simulink model "multi__micro1nosw_droop"  (R2015a)
settings: Solver=ode23tb  StartTime=0.0  StopTime=2
model workspace: external: MAT-File D:\google drive\project\nn1\matla.mat (data not in the file)
undefined symbols (not defined in the file): cf, gam, gamp, k1, k2, k3, k5, Lc, lf, mp1, mp2, Mu, nq1, nq2, rc, sig, sigp, td, wn
libraries: powerlib x113, simulink x32, powerlib_meascontrol x32, powerlib_extras x2
(part 5 of 5)

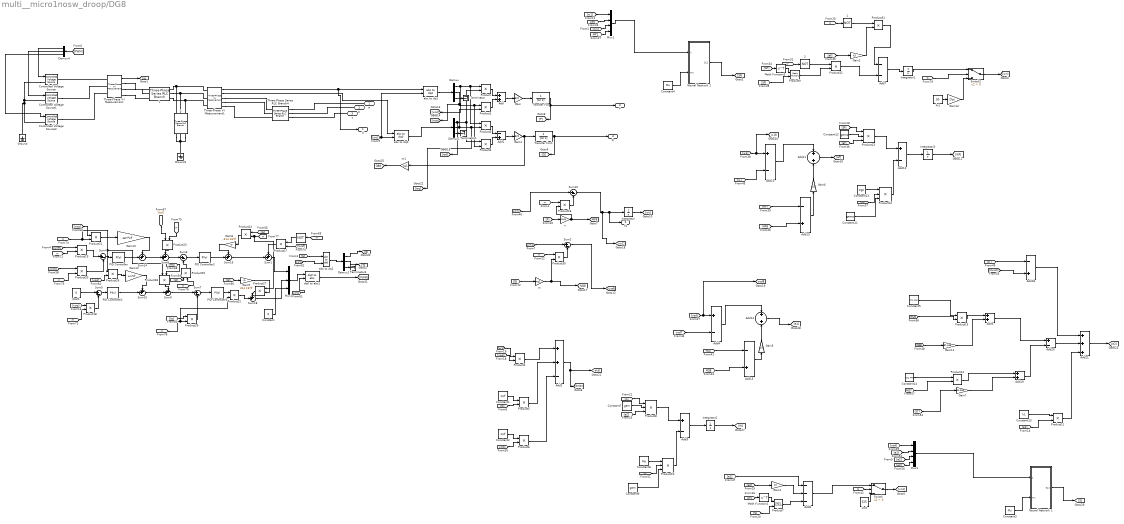
== system multi__micro1nosw_droop/DG8 ==
  " " : Logic  Operator=NOT  AllPortsSameDT=off  OutDataTypeStr=boolean
  " 1" : Logic  Operator=NOT  AllPortsSameDT=off  OutDataTypeStr=boolean
  " 2" : Logic  Operator=NOT  AllPortsSameDT=off  OutDataTypeStr=boolean
  Add{,5,11,14,19} (5 alike) : Sum
  Add{1,13,15,18} (4 alike) : Sum  Inputs=-+
  Add{4,9..10,12,20} (5 alike) : Sum  Inputs=+-
  Add2 : Sum  Inputs=++-
  Add21 : Sum  Inputs=+++
  Add7 : Sum  Inputs=--
  Add8 : Sum  Inputs=---
  C : powerlib/Elements/Three-Phase Series RLC Branch  LConnTagsString=A|B|C  RConnTagsString=A|B|C  BranchType=C  Resistance=1  Inductance=1e-3  Capacitance=cf  Measurements=None
  Constant : Constant  Value=0
  Constant1 : Constant  Value=1/cf
  Constant11 : Constant  Value=gamp
  Constant12 : Constant  Value=gamp
  Constant13 : Constant  Value=sigp
  Constant14 : Constant  Value=-31.446
  Constant15 : Constant  Value=k1
  Constant2 : Constant  Value=1/cf
  Constant3 : Constant  Value=Mu
  Constant4 : Constant  Value=Mu
  Constant5 : Constant  Value=-31.446
  Constant7 : Constant  Value=gam
  Constant8 : Constant  Value=sig
  Constant9 : Constant  Value=gam
  Controlled Voltage Source : powerlib/Electrical Sources/Controlled Voltage Source  Initialize=off  Source_Type=AC  Amplitude=325  Phase=0  Frequency=50  Measurements=None
  Controlled Voltage Source1 : powerlib/Electrical Sources/Controlled Voltage Source  Initialize=off  Source_Type=AC  Amplitude=325  Phase=0  Frequency=50  Measurements=None
  Controlled Voltage Source2 : powerlib/Electrical Sources/Controlled Voltage Source  Initialize=off  Source_Type=AC  Amplitude=325  Phase=0  Frequency=50  Measurements=None
  Demux{,1..2,4} (4 alike) : Demux  Outputs=3
  Gain : Gain  Gain=3/2
  Gain1 : Gain  Gain=3/2
  Gain10 : Gain  Gain=-wn*cf
  Gain11 : Gain  Gain=31.446
  Gain12 : Gain  Gain=wn*cf
  Gain13 : Gain  Gain=2*pi
  Gain2 : Gain  Gain=k3
  Gain4 : Gain  Gain=k2
  Gain5 : Gain  Gain=k5
  Gain6 : Gain  Gain=k5
  Gain7 : Gain  Gain=31.446
  Gain8 : Gain  Gain=-314.16*lf
  Gain9 : Gain  Gain=314.16*lf
  Ground : powerlib/Elements/Ground  LConnTagsString=a
  Ground1 : powerlib/Elements/Ground  LConnTagsString=a
  Integrator : Integrator  UpperSaturationLimit=314.16  ZeroCross=off
  Integrator1 : Integrator  InitialCondition=wn-1  UpperSaturationLimit=321  LowerSaturationLimit=314.16
  Integrator2 : Integrator  InitialCondition=zeros(16.,1)  UpperSaturationLimit=314.16  ZeroCross=off
  Integrator3 : Integrator  InitialCondition=zeros(16,1)  UpperSaturationLimit=314.16  ZeroCross=off
  L : powerlib/Elements/Three-Phase Series RLC Branch  LConnTagsString=A|B|C  RConnTagsString=A|B|C  BranchType=RL  Resistance=0.1  Inductance=lf  Capacitance=1e-6  Measurements=None
  Math Function1 : Math  Operator=transpose  OutputSignalType=real  SaturateOnIntegerOverflow=on
  Math Function3 : Math  Operator=transpose  OutputSignalType=real  SaturateOnIntegerOverflow=on
  Mux1 : Mux
  Mux2 : Mux  Inputs=3
  Mux3 : Mux
  Neural Network 1 : MATLAB Function  TreatAsAtomicUnit=on
  Neural Network 2 : MATLAB Function  TreatAsAtomicUnit=on
  PID Controller : simulink/Continuous/PID Controller  Controller=PI  TimeDomain=Continuous-time  SampleTime=-1  IntegratorMethod=Forward Euler  FilterMethod=Forward Euler  Form=Parallel  UseFilter=on  ControllerParametersSource=internal  P=0.1  I=420  D=0  N=0  InitialConditionSource=internal  InitialConditionForIntegrator=0  InitialConditionForFilter=0  ExternalReset=none  LimitOutput=off  UpperSaturationLimit=inf  LowerSaturationLimit=-inf  LinearizeAsGain=on  AntiWindupMode=none  Kb=1  TrackingMode=off  Kt=1  PParamMin=[]  PParamMax=[]  IParamMin=[]  IParamMax=[]  DParamMin=[]  DParamMax=[]  NParamMin=[]  NParamMax=[]  KbParamMin=[]  KbParamMax=[]  KtParamMin=[]  KtParamMax=[]  POutMin=[]  POutMax=[]  IOutMin=[]  IOutMax=[]  DOutMin=[]  DOutMax=[]  NOutMin=[]  NOutMax=[]  KbOutMin=[]  KbOutMax=[]  KtOutMin=[]  KtOutMax=[]  IntegratorOutMin=[]  IntegratorOutMax=[]  FilterOutMin=[]  FilterOutMax=[]  SumOutMin=[]  SumOutMax=[]  SumI1OutMin=[]  SumI1OutMax=[]  SumI2OutMin=[]  SumI2OutMax=[]  SumI3OutMin=[]  SumI3OutMax=[]  SumDOutMin=[]  SumDOutMax=[]  SaturationOutMin=[]  SaturationOutMax=[]  IntegratorContinuousStateAttributes=''  IntegratorStateMustResolveToSignalObject=off  IntegratorRTWStateStorageClass=Auto  FilterContinuousStateAttributes=''  FilterStateMustResolveToSignalObject=off  FilterRTWStateStorageClass=Auto  DifferentiatorICPrevScaledInput=0  DifferentiatorOutMin=[]  DifferentiatorOutMax=[]
  PID Controller1 : simulink/Continuous/PID Controller  Controller=PI  TimeDomain=Continuous-time  SampleTime=-1  IntegratorMethod=Forward Euler  FilterMethod=Forward Euler  Form=Parallel  UseFilter=on  ControllerParametersSource=internal  P=0.1  I=420  D=0  N=0  InitialConditionSource=internal  InitialConditionForIntegrator=0  InitialConditionForFilter=0  ExternalReset=none  LimitOutput=off  UpperSaturationLimit=inf  LowerSaturationLimit=-inf  LinearizeAsGain=on  AntiWindupMode=none  Kb=1  TrackingMode=off  Kt=1  PParamMin=[]  PParamMax=[]  IParamMin=[]  IParamMax=[]  DParamMin=[]  DParamMax=[]  NParamMin=[]  NParamMax=[]  KbParamMin=[]  KbParamMax=[]  KtParamMin=[]  KtParamMax=[]  POutMin=[]  POutMax=[]  IOutMin=[]  IOutMax=[]  DOutMin=[]  DOutMax=[]  NOutMin=[]  NOutMax=[]  KbOutMin=[]  KbOutMax=[]  KtOutMin=[]  KtOutMax=[]  IntegratorOutMin=[]  IntegratorOutMax=[]  FilterOutMin=[]  FilterOutMax=[]  SumOutMin=[]  SumOutMax=[]  SumI1OutMin=[]  SumI1OutMax=[]  SumI2OutMin=[]  SumI2OutMax=[]  SumI3OutMin=[]  SumI3OutMax=[]  SumDOutMin=[]  SumDOutMax=[]  SaturationOutMin=[]  SaturationOutMax=[]  IntegratorContinuousStateAttributes=''  IntegratorStateMustResolveToSignalObject=off  IntegratorRTWStateStorageClass=Auto  FilterContinuousStateAttributes=''  FilterStateMustResolveToSignalObject=off  FilterRTWStateStorageClass=Auto  DifferentiatorICPrevScaledInput=0  DifferentiatorOutMin=[]  DifferentiatorOutMax=[]
  PID Controller2 : simulink/Continuous/PID Controller  Controller=PI  TimeDomain=Continuous-time  SampleTime=-1  IntegratorMethod=Forward Euler  FilterMethod=Forward Euler  Form=Parallel  UseFilter=on  ControllerParametersSource=internal  P=15  I=20000  D=0  N=0  InitialConditionSource=internal  InitialConditionForIntegrator=0  InitialConditionForFilter=0  ExternalReset=none  LimitOutput=off  UpperSaturationLimit=inf  LowerSaturationLimit=-inf  LinearizeAsGain=on  AntiWindupMode=none  Kb=1  TrackingMode=off  Kt=1  PParamMin=[]  PParamMax=[]  IParamMin=[]  IParamMax=[]  DParamMin=[]  DParamMax=[]  NParamMin=[]  NParamMax=[]  KbParamMin=[]  KbParamMax=[]  KtParamMin=[]  KtParamMax=[]  POutMin=[]  POutMax=[]  IOutMin=[]  IOutMax=[]  DOutMin=[]  DOutMax=[]  NOutMin=[]  NOutMax=[]  KbOutMin=[]  KbOutMax=[]  KtOutMin=[]  KtOutMax=[]  IntegratorOutMin=[]  IntegratorOutMax=[]  FilterOutMin=[]  FilterOutMax=[]  SumOutMin=[]  SumOutMax=[]  SumI1OutMin=[]  SumI1OutMax=[]  SumI2OutMin=[]  SumI2OutMax=[]  SumI3OutMin=[]  SumI3OutMax=[]  SumDOutMin=[]  SumDOutMax=[]  SaturationOutMin=[]  SaturationOutMax=[]  IntegratorContinuousStateAttributes=''  IntegratorStateMustResolveToSignalObject=off  IntegratorRTWStateStorageClass=Auto  FilterContinuousStateAttributes=''  FilterStateMustResolveToSignalObject=off  FilterRTWStateStorageClass=Auto  DifferentiatorICPrevScaledInput=0  DifferentiatorOutMin=[]  DifferentiatorOutMax=[]
  PID Controller3 : simulink/Continuous/PID Controller  Controller=PI  TimeDomain=Continuous-time  SampleTime=-1  IntegratorMethod=Forward Euler  FilterMethod=Forward Euler  Form=Parallel  UseFilter=on  ControllerParametersSource=internal  P=15  I=20000  D=0  N=0  InitialConditionSource=internal  InitialConditionForIntegrator=0  InitialConditionForFilter=0  ExternalReset=none  LimitOutput=off  UpperSaturationLimit=inf  LowerSaturationLimit=-inf  LinearizeAsGain=on  AntiWindupMode=none  Kb=1  TrackingMode=off  Kt=1  PParamMin=[]  PParamMax=[]  IParamMin=[]  IParamMax=[]  DParamMin=[]  DParamMax=[]  NParamMin=[]  NParamMax=[]  KbParamMin=[]  KbParamMax=[]  KtParamMin=[]  KtParamMax=[]  POutMin=[]  POutMax=[]  IOutMin=[]  IOutMax=[]  DOutMin=[]  DOutMax=[]  NOutMin=[]  NOutMax=[]  KbOutMin=[]  KbOutMax=[]  KtOutMin=[]  KtOutMax=[]  IntegratorOutMin=[]  IntegratorOutMax=[]  FilterOutMin=[]  FilterOutMax=[]  SumOutMin=[]  SumOutMax=[]  SumI1OutMin=[]  SumI1OutMax=[]  SumI2OutMin=[]  SumI2OutMax=[]  SumI3OutMin=[]  SumI3OutMax=[]  SumDOutMin=[]  SumDOutMax=[]  SaturationOutMin=[]  SaturationOutMax=[]  IntegratorContinuousStateAttributes=''  IntegratorStateMustResolveToSignalObject=off  IntegratorRTWStateStorageClass=Auto  FilterContinuousStateAttributes=''  FilterStateMustResolveToSignalObject=off  FilterRTWStateStorageClass=Auto  DifferentiatorICPrevScaledInput=0  DifferentiatorOutMin=[]  DifferentiatorOutMax=[]
  Product{,1,3..4} (4 alike) : Product  RndMeth=Zero
  Product{8,10,12..13} (4 alike) : Product  Inputs=3
  Product{2,5..6,11,14..32} (23 alike) : Product
  Product7 : Product  Multiplication=Matrix(*)
  Product9 : Product  Multiplication=Matrix(*)
  Qref1 : Constant  Value=0
  Sum{1,8..9,14..16,18} (7 alike) : Sum  Inputs=++|  SaturateOnIntegerOverflow=on  InputSameDT=on  OutDataTypeStr=Inherit: Same as first input
  Sum{2,4..7,10} (6 alike) : Sum  Inputs=|+-
  Switch : Switch  Criteria=u2 > Threshold
  Switch2 : Switch  Criteria=u2 > Threshold  ZeroCross=off
  Terminator : Terminator
  Terminator1 : Terminator
  Terminator4 : Terminator
  Three-Phase Series RLC Branch4 : powerlib/Elements/Three-Phase Series RLC Branch  LConnTagsString=A|B|C  RConnTagsString=A|B|C  BranchType=RL  Resistance=rc  Inductance=Lc  Capacitance=1e-6  Measurements=None
  Three-Phase V-I Measurement : powerlib/Measurements/Three-Phase V-I Measurement  VoltageMeasurement=no  SetLabelV=off  LabelV=Vabc  Vpu=off  VpuLL=off  CurrentMeasurement=yes  SetLabelI=off  LabelI=Iabc  Ipu=off  Pbase=100e6  Vbase=500e3  OutputType=Complex  PhasorSimulation=off  PSBequivalent=0
  Three-Phase V-I Measurement1 : powerlib/Measurements/Three-Phase V-I Measurement  VoltageMeasurement=phase-to-ground  SetLabelV=off  LabelV=Vabc  Vpu=off  VpuLL=off  CurrentMeasurement=yes  SetLabelI=off  LabelI=Iabc  Ipu=off  Pbase=100e6  Vbase=500e3  OutputType=Complex  PhasorSimulation=off  PSBequivalent=0
  Transfer Fcn : TransferFcn  Denominator=[td 1]
  Transfer Fcn1 : TransferFcn  Denominator=[td 1]
  Un5 : Constant  Value=325
  abc to dq0 : powerlib_meascontrol/Transformations/abc to dq0  Alignment=90 degrees behind phase A axis
  abc to dq1 : powerlib_meascontrol/Transformations/abc to dq0  Alignment=90 degrees behind phase A axis
  abc to dq2 : powerlib_meascontrol/Transformations/abc to dq0  Alignment=90 degrees behind phase A axis
  dq0 to abc1 : powerlib_meascontrol/Transformations/dq0 to abc  Alignment=90 degrees behind phase A axis
  fn1 : Constant  Value=50
  m : Gain  Gain=nq1
  m1 : Gain  Gain=nq1
  n : Gain  Gain=mp1
  a : PMIOPort  Tag=PMCPort  Port=1  Side=Right
  b : PMIOPort  Tag=PMCPort  Port=2  Side=Right
  c : PMIOPort  Tag=PMCPort  Port=3  Side=Right
  U : Outport
  f1 : Outport  Port=2
  P : Outport  Port=3
  Q : Outport  Port=4
  tag scope: MP8=global, NQ8=global, Q88=global, dv8=global, vod8=global, w18=global
  wires:
  [PWM] -> Demux4/1
  Three-Phase V-I Measurement1/1 -> U/1, abc to dq1/1
  Three-Phase V-I Measurement1/2 -> abc to dq0/1
  Demux/1 -> [vod], Product/1, Product3/1
  Demux1/1 -> [iod], Product/2, Product4/1
  Demux/2 -> [voq], Product1/1, Product4/2
  Demux1/2 -> Product1/2, [ioq], Product3/2
  Product/1 -> Add/1
  Product1/1 -> Add/2
  Product3/1 -> Add1/1
  Product4/1 -> Add1/2
  [wt] -> abc to dq1/2, abc to dq0/2
  [P] -> n/1
  Demux4/1 -> Controlled Voltage Source/1
  Demux4/2 -> Controlled Voltage Source1/1
  Demux4/3 -> Controlled Voltage Source2/1
  Three-Phase V-I Measurement/1 -> [IL]
  Add/1 -> Gain/1
  Gain/1 -> Transfer Fcn/1
  Add1/1 -> Gain1/1
  Gain1/1 -> m1/1, Transfer Fcn1/1
  abc to dq1/1 -> Demux/1
  abc to dq0/1 -> Demux1/1
  [wn] -> Sum10/1
  Integrator/1 -> [wt]
  [w1] -> Product2/1
  [voq] -> Product2/2
  Product2/1 -> Add2/1
  Constant1/1 -> Product5/1
  [Id] -> Product5/2
  Product5/1 -> Add2/2
  Constant2/1 -> Product6/1
  [iod] -> Product6/2
  Product6/1 -> Add2/3
  Add2/1 -> [dvodi], [dv8]
  Demux/3 -> Terminator/1
  Demux1/3 -> Terminator1/1
  [Q] -> m/1
  Sum2/1 -> [Uref]
  Gain4/1 -> Add8/2
  [e2] -> Gain4/1
  [S] -> Product7/2
  [W] -> Math Function1/1
  Math Function1/1 -> Product7/1
  Product7/1 -> Add8/3
  [S] -> Product8/1
  Constant7/1 -> Product8/2
  [e2] -> Product8/3
  Product8/1 -> Add9/1
  Constant8/1 -> Product10/1
  [W] -> Product10/2
  Product10/1 -> Add9/2
  Constant9/1 -> Product10/3
  Add9/1 -> Integrator2/1
  Integrator2/1 -> [W]
  Transfer Fcn/1 -> P/1, [P]
  Transfer Fcn1/1 -> Q/1, [Q]
  [Sf] -> Product13/1
  Constant12/1 -> Product13/2
  [ef] -> Product13/3
  Product13/1 -> Add12/1
  Constant13/1 -> Product12/1
  [Wf] -> Product12/2
  Product12/1 -> Add12/2
  Constant11/1 -> Product12/3
  Add12/1 -> Integrator3/1
  Integrator3/1 -> [Wf]
  [w1] -> Mux1/1
  [ef] -> Mux1/2
  [wn] -> Mux1/3
  [MP1] -> Mux1/4
  [w1] -> [w18], Add10/1
  [w17] -> Add10/2
  Add10/1 -> Add11/1
  [MP7] -> Add13/1
  [MP8] -> Add13/2
  Add13/1 -> Gain6/1
  Add11/1 -> [ef]
  [vod] -> [vod8], Add4/1
  [vod7] -> Add4/2
  Add4/1 -> Add14/1
  [NQ7] -> Add15/1
  [NQ8] -> Add15/2
  Add15/1 -> Gain5/1
  Add14/1 -> [e1]
  Gain5/1 -> Add14/2
  Gain6/1 -> Add11/2
  [e1] -> Add8/1
  m1/1 -> [Q88]
  [vod] -> Mux3/1
  [e1] -> Mux3/2
  [e2] -> Mux3/3
  [e2] -> Mux3/4
  Constant5/1 -> Product15/1
  [NQ8] -> Product15/2
  Product15/1 -> Add5/1
  [Q88] -> Gain11/1
  Constant14/1 -> Product14/1
  [NQ7] -> Product14/2
  Product14/1 -> Add19/1
  [Q77] -> Gain7/1
  Add19/1 -> Add20/2
  Add5/1 -> Add20/1
  Gain7/1 -> Add19/2
  Gain11/1 -> Add5/2
  Add20/1 -> Add21/2
  Constant15/1 -> Product11/1
  [e1] -> Product11/2
  Product11/1 -> Add21/3
  [dv7] -> Add18/1
  Add18/1 -> Add21/1
  Add21/1 -> [e2]
  [dvodi] -> Add18/2
  [IL] -> abc to dq2/1
  Demux2/1 -> [Id]
  Demux2/2 -> [Iq]
  [wt] -> abc to dq2/2
  Qref1/1 -> Sum5/1
  Sum4/1 -> PID Controller/1
  Sum5/1 -> PID Controller1/1
  Sum18/1 -> Mux2/2
  Constant/1 -> Mux2/3
  PID Controller/1 -> Sum14/2
  PID Controller1/1 -> Sum15/2
  Gain10/1 -> Sum14/1
  Gain12/1 -> Sum15/1
  Sum15/1 -> Sum9/2
  Sum9/1 -> Sum7/1
  Sum14/1 -> Sum8/2
  Sum8/1 -> Sum6/1
  Sum6/1 -> PID Controller2/1
  Sum7/1 -> PID Controller3/1
  Gain8/1 -> Sum16/1
  PID Controller2/1 -> Sum16/2
  [Id] -> Gain9/1
  Mux2/1 -> dq0 to abc1/1
  [wt] -> dq0 to abc1/2
  abc to dq2/1 -> Demux2/1
  dq0 to abc1/1 -> [PWM]
  Demux2/3 -> Terminator4/1
  Sum16/1 -> Sum1/2
  Sum1/1 -> Mux2/1
  Product17/1 -> Sum1/1
  [rr] -> " "/1
  [Uref] -> Product17/2
  " "/1 -> Product17/1
  [voq] -> Product18/1
  Product18/1 -> Sum5/2
  [rr] -> Product18/2
  [Uref] -> Product19/1
  Product19/1 -> Sum4/1
  [rr] -> Product19/2
  [vod] -> Product20/1
  Product20/1 -> Sum4/2
  [rr] -> Product20/2
  Product21/1 -> Gain10/1
  [voq] -> Product21/1
  [rr] -> Product28/1, Product26/1, Product21/2
  [iod] -> Product23/1
  [rr] -> Product23/2
  Product23/1 -> Sum8/1
  [Id] -> Product25/1
  Product25/1 -> Sum6/2
  [rr] -> Product25/2
  Product24/1 -> Gain8/1
  [Iq] -> Product24/1
  [rr] -> Product27/1, Product24/2
  [vod] -> Product26/2
  Product26/1 -> Gain12/1
  [ioq] -> Product28/2
  Product28/1 -> Sum9/1
  [Iq] -> Product29/1
  Product29/1 -> Sum7/2
  [rr] -> Product22/2, Product29/2
  Product27/1 -> Sum18/1
  Gain9/1 -> Product27/2
  PID Controller3/1 -> Product22/1
  Product22/1 -> Sum18/2
  [ti] -> Switch/2
  Un5/1 -> Switch/3
  Add8/1 -> Switch/1
  Switch/1 -> [vn1]
  n/1 -> [MP8], Product16/2
  Product16/1 -> Sum10/2
  [rr] -> Product16/1
  Sum10/1 -> [w1], f1/1, Integrator/1
  m/1 -> Product30/2, [NQ8]
  Product30/1 -> Sum2/2
  [rr] -> Product30/1
  [vn1] -> Sum2/1
  [Sf] -> Product9/2
  [Wf] -> Math Function3/1
  Math Function3/1 -> Product9/1
  Add7/1 -> Integrator1/1
  [ti] -> Switch2/2
  Gain13/1 -> Switch2/3
  Switch2/1 -> [wn]
  fn1/1 -> Gain13/1
  [ef] -> Gain2/1
  [rr] -> " 1"/1
  Gain2/1 -> Product31/2
  " 1"/1 -> Product31/1
  Product31/1 -> Add7/1
  [rr] -> " 2"/1
  Product9/1 -> Product32/2
  " 2"/1 -> Product32/1
  Product32/1 -> Add7/2
  Integrator1/1 -> Switch2/1
  Neural Network 1/1(Sz1) -> [S]
  Constant3/1 -> Neural Network 1/2(mu)
  Mux3/1 -> Neural Network 1/1(X)
  Neural Network 2/1(Sz1) -> [Sf]
  Constant4/1 -> Neural Network 2/2(mu)
  Mux1/1 -> Neural Network 2/1(X)
  connections:
  C/RConn1 -- Ground1/LConn1 -- C/RConn3 -- C/RConn2
  L/RConn2 -- Three-Phase V-I Measurement1/LConn2 -- C/LConn2
  L/RConn1 -- Three-Phase V-I Measurement1/LConn1 -- C/LConn1
  L/RConn3 -- Three-Phase V-I Measurement1/LConn3 -- C/LConn3
  Controlled Voltage Source/LConn1 -- Controlled Voltage Source1/LConn1 -- Ground/LConn1 -- Controlled Voltage Source2/LConn1
  Three-Phase V-I Measurement/LConn1 -- Controlled Voltage Source/RConn1
  Controlled Voltage Source1/RConn1 -- Three-Phase V-I Measurement/LConn2
  Controlled Voltage Source2/RConn1 -- Three-Phase V-I Measurement/LConn3
  Three-Phase V-I Measurement/RConn1 -- L/LConn1
  Three-Phase V-I Measurement/RConn2 -- L/LConn2
  Three-Phase V-I Measurement/RConn3 -- L/LConn3
  Three-Phase V-I Measurement1/RConn1 -- Three-Phase Series RLC Branch4/RConn1
  Three-Phase V-I Measurement1/RConn2 -- Three-Phase Series RLC Branch4/RConn2
  Three-Phase V-I Measurement1/RConn3 -- Three-Phase Series RLC Branch4/RConn3
  Three-Phase Series RLC Branch4/LConn1 -- a/RConn1
  Three-Phase Series RLC Branch4/LConn2 -- b/RConn1
  Three-Phase Series RLC Branch4/LConn3 -- c/RConn1

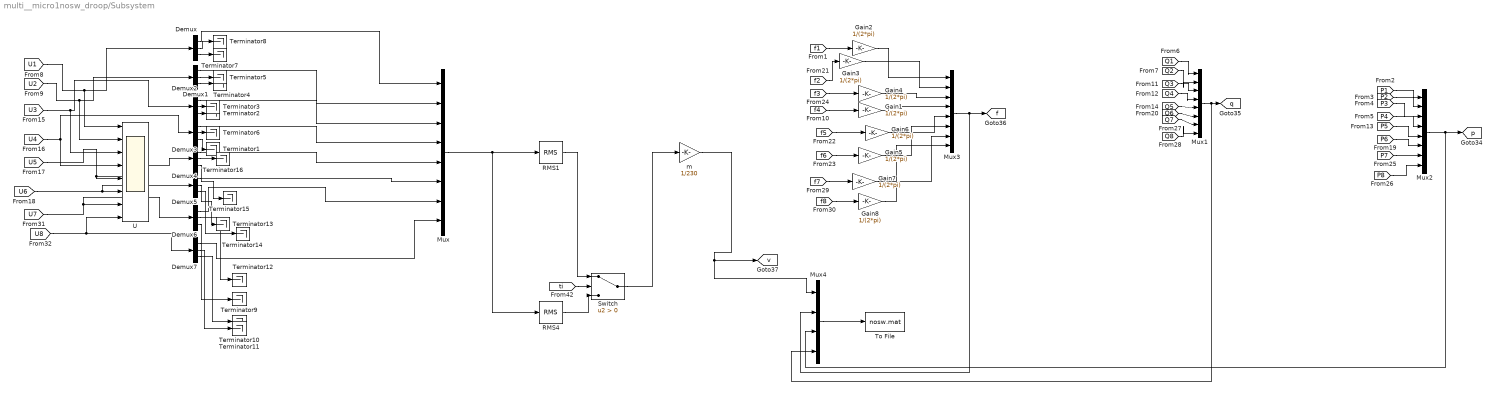
== system multi__micro1nosw_droop/Subsystem ==
  Demux{,1..7} (8 alike) : Demux  Outputs=3
  Gain{1..8} (8 alike) : Gain  Gain=1/(2*pi)
  Mux{,1..3} (4 alike) : Mux  Inputs=8
  Mux4 : Mux
  RMS1 : powerlib_extras/Measurements/RMS  f1=50
  RMS4 : powerlib_extras/Measurements/RMS  f1=49.75
  Switch : Switch  Criteria=u2 > Threshold
  Terminator{1..16} (16 alike) : Terminator
  To File : ToFile  Filename=nosw.mat  MatrixName=case1  SaveFormat=Timeseries
  U : Scope  NumInputPorts=8
      settings: TimeRange=1  YMin=-400~-400~-400~-1~-1~-1~-1~-1  YMax=400~400~400~1~1~1~1~1  SaveName=U
  m : Gain  Gain=1/230
  tag scope: f=global, p=global, q=global, v=global
  wires:
  [U6] -> Demux5/1, U/6
  Demux3/3 -> Terminator1/1
  Demux2/1 -> Mux/3
  [U5] -> Demux4/1, U/5
  Demux3/2 -> Terminator6/1
  Demux1/1 -> Mux/2
  [U4] -> Demux3/1, U/4
  Demux3/1 -> Mux/4
  Demux4/1 -> Mux/5
  Demux5/1 -> Mux/6
  Demux/3 -> Terminator7/1
  Demux2/2 -> Terminator3/1
  Demux1/3 -> Terminator4/1
  Demux1/2 -> Terminator5/1
  [U2] -> Demux1/1, U/2
  Demux/2 -> Terminator8/1
  [U3] -> Demux2/1, U/3
  [U1] -> Demux/1, U/1
  Demux2/3 -> Terminator2/1
  [U7] -> U/7, Demux6/1
  Demux7/1 -> Mux/8
  Demux6/2 -> Terminator12/1
  Demux6/3 -> Terminator9/1
  Demux5/2 -> Terminator13/1
  Demux7/2 -> Terminator11/1
  Demux4/3 -> Terminator15/1
  Demux5/3 -> Terminator14/1
  [U8] -> Demux7/1, U/8
  Demux7/3 -> Terminator10/1
  Demux4/2 -> Terminator16/1
  m/1 -> Mux4/1, [v]
  [f4] -> Gain1/1
  [f1] -> Gain2/1
  Gain1/1 -> Mux3/4
  [f3] -> Gain4/1
  [f5] -> Gain6/1
  [f6] -> Gain5/1
  Gain2/1 -> Mux3/1
  [f2] -> Gain3/1
  Gain3/1 -> Mux3/2
  Gain4/1 -> Mux3/3
  Gain5/1 -> Mux3/6
  Gain6/1 -> Mux3/5
  [f7] -> Gain7/1
  Gain7/1 -> Mux3/7
  [f8] -> Gain8/1
  Gain8/1 -> Mux3/8
  Mux3/1 -> Mux4/2, [f]
  [Q1] -> Mux1/1
  [Q3] -> Mux1/3
  [Q2] -> Mux1/2
  [Q4] -> Mux1/4
  [Q5] -> Mux1/5
  [Q6] -> Mux1/6
  [Q7] -> Mux1/7
  [Q8] -> Mux1/8
  Mux1/1 -> Mux4/4, [q]
  [P2] -> Mux2/2
  [P1] -> Mux2/1
  [P3] -> Mux2/3
  [P4] -> Mux2/4
  [P5] -> Mux2/5
  [P6] -> Mux2/6
  [P7] -> Mux2/7
  [P8] -> Mux2/8
  Mux2/1 -> Mux4/3, [p]
  Mux4/1 -> To File/1
  Demux/1 -> Mux/1
  Demux6/1 -> Mux/7
  [ti] -> Switch/2
  RMS4/1 -> Switch/3
  RMS1/1 -> Switch/1
  Mux/1 -> RMS1/1, RMS4/1
  Switch/1 -> m/1

== matlab function multi__micro1nosw_droop/DG1/Neural Network 2 ==
  settings: fimath=|
      | fimath(...
      | 'RoundMode', 'floor',...
      | 'OverflowMode', 'wrap',...
      | 'ProductMode', 'KeepLSB', 'ProductWordLength', 32,...
      | 'SumMode', 'KeepLSB', 'SumWordLength', 32,...
      | 'CastBeforeSum', false)
  data: Sz1 output; X input; mu input


function Sz1 =NNappr(X,mu)

Sz1=zeros(16,1);
for i=1:16
   Sz1(i,1)=exp(-transpose(X-mu(:,i))*(X-mu(:,i))/(10^2));   
end

== matlab function multi__micro1nosw_droop/DG2/Neural Network 1 ==
  settings: fimath=|
      | fimath(...
      | 'RoundMode', 'floor',...
      | 'OverflowMode', 'wrap',...
      | 'ProductMode', 'KeepLSB', 'ProductWordLength', 32,...
      | 'SumMode', 'KeepLSB', 'SumWordLength', 32,...
      | 'CastBeforeSum', false)
  data: Sz1 output; X input; mu input


function Sz1 =NNappr(X,mu)

Sz1=zeros(16,1);
for i=1:16
   Sz1(i,1)=exp(-transpose(X-mu(:,i))*(X-mu(:,i))/(10^2));   
end

== matlab function multi__micro1nosw_droop/DG2/Neural Network 2 ==
  settings: fimath=|
      | fimath(...
      | 'RoundMode', 'floor',...
      | 'OverflowMode', 'wrap',...
      | 'ProductMode', 'KeepLSB', 'ProductWordLength', 32,...
      | 'SumMode', 'KeepLSB', 'SumWordLength', 32,...
      | 'CastBeforeSum', false)
  data: Sz1 output; X input; mu input


function Sz1 =NNappr(X,mu)

Sz1=zeros(16,1);
for i=1:16
   Sz1(i,1)=exp(-transpose(X-mu(:,i))*(X-mu(:,i))/(10^2));   
end

== matlab function multi__micro1nosw_droop/DG1/Neural Network 1 ==
  settings: fimath=|
      | fimath(...
      | 'RoundMode', 'floor',...
      | 'OverflowMode', 'wrap',...
      | 'ProductMode', 'KeepLSB', 'ProductWordLength', 32,...
      | 'SumMode', 'KeepLSB', 'SumWordLength', 32,...
      | 'CastBeforeSum', false)
  data: Sz1 output; X input; mu input


function Sz1 =NNappr(X,mu)

Sz1=zeros(16,1);
for i=1:16
   Sz1(i,1)=exp(-transpose(X-mu(:,i))*(X-mu(:,i))/(10^2));   
end

== matlab function multi__micro1nosw_droop/DG3/Neural Network 1 ==
  settings: fimath=|
      | fimath(...
      | 'RoundMode', 'floor',...
      | 'OverflowMode', 'wrap',...
      | 'ProductMode', 'KeepLSB', 'ProductWordLength', 32,...
      | 'SumMode', 'KeepLSB', 'SumWordLength', 32,...
      | 'CastBeforeSum', false)
  data: Sz1 output; X input; mu input


function Sz1 =NNappr(X,mu)

Sz1=zeros(16,1);
for i=1:16
   Sz1(i,1)=exp(-transpose(X-mu(:,i))*(X-mu(:,i))/(10^2));   
end

== matlab function multi__micro1nosw_droop/DG3/Neural Network 2 ==
  settings: fimath=|
      | fimath(...
      | 'RoundMode', 'floor',...
      | 'OverflowMode', 'wrap',...
      | 'ProductMode', 'KeepLSB', 'ProductWordLength', 32,...
      | 'SumMode', 'KeepLSB', 'SumWordLength', 32,...
      | 'CastBeforeSum', false)
  data: Sz1 output; X input; mu input


function Sz1 =NNappr(X,mu)

Sz1=zeros(16,1);
for i=1:16
   Sz1(i,1)=exp(-transpose(X-mu(:,i))*(X-mu(:,i))/(10^2));   
end

== matlab function multi__micro1nosw_droop/DG4/Neural Network 1 ==
  settings: fimath=|
      | fimath(...
      | 'RoundMode', 'floor',...
      | 'OverflowMode', 'wrap',...
      | 'ProductMode', 'KeepLSB', 'ProductWordLength', 32,...
      | 'SumMode', 'KeepLSB', 'SumWordLength', 32,...
      | 'CastBeforeSum', false)
  data: Sz1 output; X input; mu input


function Sz1 =NNappr(X,mu)

Sz1=zeros(16,1);
for i=1:16
   Sz1(i,1)=exp(-transpose(X-mu(:,i))*(X-mu(:,i))/(10^2));   
end

== matlab function multi__micro1nosw_droop/DG4/Neural Network 2 ==
  settings: fimath=|
      | fimath(...
      | 'RoundMode', 'floor',...
      | 'OverflowMode', 'wrap',...
      | 'ProductMode', 'KeepLSB', 'ProductWordLength', 32,...
      | 'SumMode', 'KeepLSB', 'SumWordLength', 32,...
      | 'CastBeforeSum', false)
  data: Sz1 output; X input; mu input


function Sz1 =NNappr(X,mu)

Sz1=zeros(16,1);
for i=1:16
   Sz1(i,1)=exp(-transpose(X-mu(:,i))*(X-mu(:,i))/(10^2));   
end

== matlab function multi__micro1nosw_droop/DG5/Neural Network 1 ==
  settings: fimath=|
      | fimath(...
      | 'RoundMode', 'floor',...
      | 'OverflowMode', 'wrap',...
      | 'ProductMode', 'KeepLSB', 'ProductWordLength', 32,...
      | 'SumMode', 'KeepLSB', 'SumWordLength', 32,...
      | 'CastBeforeSum', false)
  data: Sz1 output; X input; mu input


function Sz1 =NNappr(X,mu)

Sz1=zeros(16,1);
for i=1:16
   Sz1(i,1)=exp(-transpose(X-mu(:,i))*(X-mu(:,i))/(10^2));   
end

== matlab function multi__micro1nosw_droop/DG5/Neural Network 2 ==
  settings: fimath=|
      | fimath(...
      | 'RoundMode', 'floor',...
      | 'OverflowMode', 'wrap',...
      | 'ProductMode', 'KeepLSB', 'ProductWordLength', 32,...
      | 'SumMode', 'KeepLSB', 'SumWordLength', 32,...
      | 'CastBeforeSum', false)
  data: Sz1 output; X input; mu input


function Sz1 =NNappr(X,mu)

Sz1=zeros(16,1);
for i=1:16
   Sz1(i,1)=exp(-transpose(X-mu(:,i))*(X-mu(:,i))/(10^2));   
end

== matlab function multi__micro1nosw_droop/DG6/Neural Network 1 ==
  settings: fimath=|
      | fimath(...
      | 'RoundMode', 'floor',...
      | 'OverflowMode', 'wrap',...
      | 'ProductMode', 'KeepLSB', 'ProductWordLength', 32,...
      | 'SumMode', 'KeepLSB', 'SumWordLength', 32,...
      | 'CastBeforeSum', false)
  data: Sz1 output; X input; mu input


function Sz1 =NNappr(X,mu)

Sz1=zeros(16,1);
for i=1:16
   Sz1(i,1)=exp(-transpose(X-mu(:,i))*(X-mu(:,i))/(10^2));   
end

== matlab function multi__micro1nosw_droop/DG6/Neural Network 2 ==
  settings: fimath=|
      | fimath(...
      | 'RoundMode', 'floor',...
      | 'OverflowMode', 'wrap',...
      | 'ProductMode', 'KeepLSB', 'ProductWordLength', 32,...
      | 'SumMode', 'KeepLSB', 'SumWordLength', 32,...
      | 'CastBeforeSum', false)
  data: Sz1 output; X input; mu input


function Sz1 =NNappr(X,mu)

Sz1=zeros(16,1);
for i=1:16
   Sz1(i,1)=exp(-transpose(X-mu(:,i))*(X-mu(:,i))/(10^2));   
end

== matlab function multi__micro1nosw_droop/DG7/Neural Network 1 ==
  settings: fimath=|
      | fimath(...
      | 'RoundMode', 'floor',...
      | 'OverflowMode', 'wrap',...
      | 'ProductMode', 'KeepLSB', 'ProductWordLength', 32,...
      | 'SumMode', 'KeepLSB', 'SumWordLength', 32,...
      | 'CastBeforeSum', false)
  data: Sz1 output; X input; mu input


function Sz1 =NNappr(X,mu)

Sz1=zeros(16,1);
for i=1:16
   Sz1(i,1)=exp(-transpose(X-mu(:,i))*(X-mu(:,i))/(10^2));   
end

== matlab function multi__micro1nosw_droop/DG7/Neural Network 2 ==
  settings: fimath=|
      | fimath(...
      | 'RoundMode', 'floor',...
      | 'OverflowMode', 'wrap',...
      | 'ProductMode', 'KeepLSB', 'ProductWordLength', 32,...
      | 'SumMode', 'KeepLSB', 'SumWordLength', 32,...
      | 'CastBeforeSum', false)
  data: Sz1 output; X input; mu input


function Sz1 =NNappr(X,mu)

Sz1=zeros(16,1);
for i=1:16
   Sz1(i,1)=exp(-transpose(X-mu(:,i))*(X-mu(:,i))/(10^2));   
end

== matlab function multi__micro1nosw_droop/DG8/Neural Network 1 ==
  settings: fimath=|
      | fimath(...
      | 'RoundMode', 'floor',...
      | 'OverflowMode', 'wrap',...
      | 'ProductMode', 'KeepLSB', 'ProductWordLength', 32,...
      | 'SumMode', 'KeepLSB', 'SumWordLength', 32,...
      | 'CastBeforeSum', false)
  data: Sz1 output; X input; mu input


function Sz1 =NNappr(X,mu)

Sz1=zeros(16,1);
for i=1:16
   Sz1(i,1)=exp(-transpose(X-mu(:,i))*(X-mu(:,i))/(10^2));   
end

== matlab function multi__micro1nosw_droop/DG8/Neural Network 2 ==
  settings: fimath=|
      | fimath(...
      | 'RoundMode', 'floor',...
      | 'OverflowMode', 'wrap',...
      | 'ProductMode', 'KeepLSB', 'ProductWordLength', 32,...
      | 'SumMode', 'KeepLSB', 'SumWordLength', 32,...
      | 'CastBeforeSum', false)
  data: Sz1 output; X input; mu input


function Sz1 =NNappr(X,mu)

Sz1=zeros(16,1);
for i=1:16
   Sz1(i,1)=exp(-transpose(X-mu(:,i))*(X-mu(:,i))/(10^2));   
end
